simulink model "ctrl_custom_4corner_automatic"  (R2016b)
settings: Solver=ode4  StartTime=0.0  StopTime=inf  FixedStep=0.01  RelTol=1e-3  EnableMultiTasking=on
values from neighbouring files (symbols this model uses):
  alpha = R_T*Eta_t_dot - K1*z_1    [Immersion.m]
undefined symbols (not defined in the file or in its folder): T_pinv_m
libraries: marine_gnc x6, simulink x1
(part 1 of 5)
settings Model: Creator=mclab  LastModifiedBy=utente
settings DataIOCC: LimitDataPoints=on  SaveFormat=Array
settings OptimizationCC: LifeSpan=inf
settings DebuggingCC: SolverPrmCheckMsg=warning  InheritedTsInSrcMsg=none  RootOutportRequireBusObject=error  StrictBusMsg=ErrorOnBusTreatedAsVector  SFUnexpectedBacktrackingDiag=warning  SFNoUnconditionalDefaultTransitionDiag=warning  SFExecutionAtInitializationDiag=none
settings HardwareCC: ProdBitPerPointer=32  ProdBitPerSizeT=32  ProdBitPerPtrDiffT=32  ProdLargestAtomicFloat=None  ProdIntDivRoundTo=Undefined  ProdEndianess=Unspecified  ProdWordSize=32  ProdHWDeviceType=32-bit Generic
settings ModelReferenceCC: PropagateSignalLabelsOutOfModel=off
settings RTWCC: SystemTargetFile=NIVeriStand_VxWorks.tlc  TemplateMakefile=NIVeriStand_VxWorks.tmf  Description=NI VeriStand VxWorks Real-Time Target for Release 2007b or later
settings STFCustomTargetCC: GeneratePreprocessorConditionals=Disable all  MatFileLogging=on  MATLABClassNameForMDSCustomization=Simulink.SoftwareTarget.TargetSpecificTriggerConfigurationBase  SystemTargetFile=NIVeriStand_VxWorks.tlc
settings ConfigComp: CovMetricSettings=dw  CovHtmlReporting=on  CovSaveCumulativeToWorkspaceVar=on  CovSaveSingleToWorkspaceVar=on  CovExternalEMLEnable=off  CovSFcnEnable=off

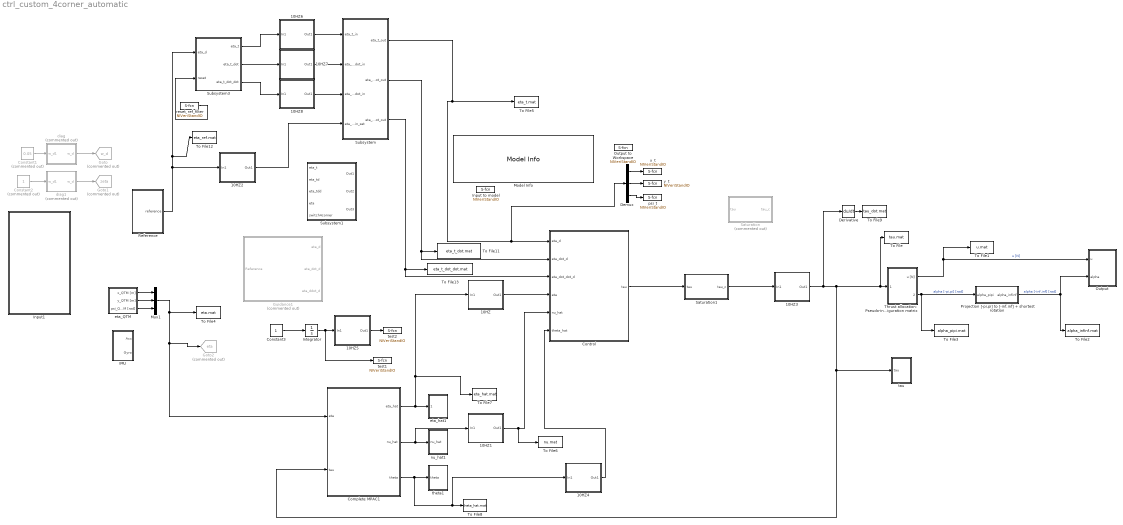
== system ctrl_custom_4corner_automatic ==
  10HZ : Subsystem
  10HZ1 : Subsystem
  10HZ2 : Subsystem
  10HZ3 : Subsystem
  10HZ4 : Subsystem
  10HZ5 : Subsystem
  10HZ6 : Subsystem
  10HZ7 : Subsystem
  10HZ8 : Subsystem
  Complete MPAC1 : Subsystem
  Constant1 : Constant  Commented=on  Value=0.05
  Constant2 : Constant  Commented=on
  Constant3 : Constant
  Control : Subsystem
  Demux : Demux  Outputs=3
  Derivative : Derivative
  Goto : Goto  Commented=on  GotoTag=w_d  TagVisibility=global
  Goto1 : Goto  Commented=on  GotoTag=zeta  TagVisibility=global
  Goto2 : Goto  Commented=on  GotoTag=eta  TagVisibility=global
  Guidance1 : Subsystem  Commented=on
  IMU : Subsystem
  Input to model : S-Function  Priority=1  FunctionName=NIVeriStandIO  Parameters=width dtype portnum stime stype btype  SFunctionDeploymentMode=off  EnableBusSupport=off  mask(NI VeriStand Inport){portnum=1, width=-1, stime=-1, dtype=auto, stype=auto, btype=1}
      mask prompts: portnum "Port number:"; width "Port dimensions (-1 for dynamically sized):"; stime "Sample time (-1 for inherited):"; dtype "Data type:"; stype "Signal type:"; btype "Block type:"
      mask help: Use this inport on any level of nested subsystems to allow NI VeriStand software to map signals to it.
      mask init:
      | NIVeriStandIO_init;
      settings: CopyFcn=NIVeriStand_MDL_functions('', 'IO_copy');  DeleteFcn=NIVeriStand_MDL_functions('', 'IO_delete');  MoveFcn=set_param(gcb, 'Mask', 'on');
      mask Callback portnum: NIVeriStand_MDL_functions('', 'IO_setportnum');
      mask TypeOptions dtype: auto | double | single | int8 | uint8 | int16 | uint16 | int32 | uint32 | boolean
      mask Callback dtype: NIVeriStand_MDL_functions('', 'IO_booleansignal');
      mask TypeOptions stype: auto | real | complex
      mask Display:
      | patch([-x x], [-y y], [.90980 .81960 .32156]);
      | plot([xrad -x x xrad], [yrad -y y yrad]);
      | fprintf('NI In%d', portnum);
  Input1 : Subsystem
  Integrator : Integrator
  Model Info : simulink/Model-Wide Utilities/Model Info  Frame=on  DisplayStringWithTags=|  HorizontalTextAlignment=Center  LeftAlignmentValue=0.5  SourceBlockDiagram=ctrl_custom  TagMaxNumber=20
      | Read me: 
      | In this model you find all the inputs and outputs for controlling CSAD. 
      | DO NOT alter the subsystems IMU, Pose or u. 
      | 
      | For real-time control (e.g. tuning controller gains when the vessel is running) 
      | and monitoring of variables, use NI Veristand Input/Output ports. 
      | You can add as many as you want. Note that these only operates on 
      | single variables, therefore use Mux/Demux/Selector.
      | These variables are accesible from VeriStand Workspace
  Mux1 : Mux  Inputs=3
  Output : Subsystem
  Output to Workspace : S-Function  Priority=1  FunctionName=NIVeriStandIO  Parameters=width dtype portnum stime stype btype  SFunctionDeploymentMode=off  EnableBusSupport=off  mask(NI VeriStand Outport){portnum=1, width=-1, stime=-1, dtype=auto, stype=auto, btype=0}
      mask prompts: portnum "Port number:"; width "Port dimensions (-1 for dynamically sized):"; stime "Sample time (-1 for inherited):"; dtype "Data type:"; stype "Signal type:"; btype "Block type:"
      mask help: Use this outport on any level of nested subsystems to allow NI VeriStand software to map signals to it.
      mask init:
      | NIVeriStandIO_init;
      settings: CopyFcn=NIVeriStand_MDL_functions('', 'IO_copy');  DeleteFcn=NIVeriStand_MDL_functions('', 'IO_delete');  MoveFcn=set_param(gcb, 'Mask', 'on');
      mask Callback portnum: NIVeriStand_MDL_functions('', 'IO_setportnum');
      mask TypeOptions dtype: auto | double | single | int8 | uint8 | int16 | uint16 | int32 | uint32 | boolean
      mask Callback dtype: NIVeriStand_MDL_functions('', 'IO_booleansignal');
      mask TypeOptions stype: auto | real | complex
      mask Display:
      | patch([-x x], [-y y], [.90980 .81960 .32156]);
      | plot([xrad -x x xrad], [yrad -y y yrad]);
      | fprintf('NI Out%d', portnum);
  Projection [-pi,pi] to [-inf,inf] + shortest rotation : Subsystem
  Reference : Subsystem
  Saturation : Subsystem  Commented=on
  Saturation1 : Subsystem
  Subsystem : Subsystem
  Subsystem1 : Subsystem
  Subsystem3 : Subsystem
  Thrust allocation: Pseudo-inverse of extended thrust configuration matrix : Subsystem
  To File : ToFile  Filename=tau.mat  MatrixName=tau
  To File1 : ToFile  Filename=u.mat
  To File11 : ToFile  Filename=eta_t_dot.mat
  To File12 : ToFile  Filename=eta_ref.mat  MatrixName=eta_t
  To File13 : ToFile  Filename=eta_t_dot_dot.mat
  To File2 : ToFile  Filename=alpha_infinf.mat
  To File3 : ToFile  Filename=alpha_pipi.mat
  To File4 : ToFile  Filename=eta.mat  MatrixName=eta
  To File5 : ToFile  Filename=eta_t.mat
  To File6 : ToFile  Filename=nu.mat  MatrixName=nu
  To File7 : ToFile  Filename=eta_hat.mat
  To File8 : ToFile  Filename=theta_hat.mat
  To File9 : ToFile  Filename=tau_dot.mat  MatrixName=tau_dot
  diag : MATLAB Function  Commented=on  TreatAsAtomicUnit=on
  diag1 : MATLAB Function  Commented=on  TreatAsAtomicUnit=on
  eta_QTM : Subsystem
  eta_hat1 : Subsystem
  nu_hat1 : Subsystem
  psi_t : S-Function  Priority=4  FunctionName=NIVeriStandIO  Parameters=width dtype portnum stime stype btype  SFunctionDeploymentMode=off  EnableBusSupport=off  mask(NI VeriStand Outport){portnum=4, width=-1, stime=-1, dtype=auto, stype=auto, btype=0}
      mask prompts: portnum "Port number:"; width "Port dimensions (-1 for dynamically sized):"; stime "Sample time (-1 for inherited):"; dtype "Data type:"; stype "Signal type:"; btype "Block type:"
      mask help: Use this outport on any level of nested subsystems to allow NI VeriStand software to map signals to it.
      mask init:
      | NIVeriStandIO_init;
      settings: CopyFcn=NIVeriStand_MDL_functions('', 'IO_copy');  DeleteFcn=NIVeriStand_MDL_functions('', 'IO_delete');  MoveFcn=set_param(gcb, 'Mask', 'on');
      mask Callback portnum: NIVeriStand_MDL_functions('', 'IO_setportnum');
      mask TypeOptions dtype: auto | double | single | int8 | uint8 | int16 | uint16 | int32 | uint32 | boolean
      mask Callback dtype: NIVeriStand_MDL_functions('', 'IO_booleansignal');
      mask TypeOptions stype: auto | real | complex
      mask Display:
      | patch([-x x], [-y y], [.90980 .81960 .32156]);
      | plot([xrad -x x xrad], [yrad -y y yrad]);
      | fprintf('NI Out%d', portnum);
  reset_ref_filter : S-Function  Priority=2  FunctionName=NIVeriStandIO  Parameters=width dtype portnum stime stype btype  SFunctionDeploymentMode=off  EnableBusSupport=off  mask(NI VeriStand Inport){portnum=2, width=-1, stime=-1, dtype=auto, stype=auto, btype=1}
      mask prompts: portnum "Port number:"; width "Port dimensions (-1 for dynamically sized):"; stime "Sample time (-1 for inherited):"; dtype "Data type:"; stype "Signal type:"; btype "Block type:"
      mask help: Use this inport on any level of nested subsystems to allow NI VeriStand software to map signals to it.
      mask init:
      | NIVeriStandIO_init;
      settings: CopyFcn=NIVeriStand_MDL_functions('', 'IO_copy');  DeleteFcn=NIVeriStand_MDL_functions('', 'IO_delete');  MoveFcn=set_param(gcb, 'Mask', 'on');
      mask Callback portnum: NIVeriStand_MDL_functions('', 'IO_setportnum');
      mask TypeOptions dtype: auto | double | single | int8 | uint8 | int16 | uint16 | int32 | uint32 | boolean
      mask Callback dtype: NIVeriStand_MDL_functions('', 'IO_booleansignal');
      mask TypeOptions stype: auto | real | complex
      mask Display:
      | patch([-x x], [-y y], [.90980 .81960 .32156]);
      | plot([xrad -x x xrad], [yrad -y y yrad]);
      | fprintf('NI In%d', portnum);
  tau : Subsystem
  test1 : S-Function  Priority=6  FunctionName=NIVeriStandIO  Parameters=width dtype portnum stime stype btype  SFunctionDeploymentMode=off  EnableBusSupport=off  mask(NI VeriStand Outport){portnum=6, width=-1, stime=-1, dtype=auto, stype=auto, btype=0}
      mask prompts: portnum "Port number:"; width "Port dimensions (-1 for dynamically sized):"; stime "Sample time (-1 for inherited):"; dtype "Data type:"; stype "Signal type:"; btype "Block type:"
      mask help: Use this outport on any level of nested subsystems to allow NI VeriStand software to map signals to it.
      mask init:
      | NIVeriStandIO_init;
      settings: CopyFcn=NIVeriStand_MDL_functions('', 'IO_copy');  DeleteFcn=NIVeriStand_MDL_functions('', 'IO_delete');  MoveFcn=set_param(gcb, 'Mask', 'on');
      mask Callback portnum: NIVeriStand_MDL_functions('', 'IO_setportnum');
      mask TypeOptions dtype: auto | double | single | int8 | uint8 | int16 | uint16 | int32 | uint32 | boolean
      mask Callback dtype: NIVeriStand_MDL_functions('', 'IO_booleansignal');
      mask TypeOptions stype: auto | real | complex
      mask Display:
      | patch([-x x], [-y y], [.90980 .81960 .32156]);
      | plot([xrad -x x xrad], [yrad -y y yrad]);
      | fprintf('NI Out%d', portnum);
  test2 : S-Function  Priority=5  FunctionName=NIVeriStandIO  Parameters=width dtype portnum stime stype btype  SFunctionDeploymentMode=off  EnableBusSupport=off  mask(NI VeriStand Outport){portnum=5, width=-1, stime=-1, dtype=auto, stype=auto, btype=0}
      mask prompts: portnum "Port number:"; width "Port dimensions (-1 for dynamically sized):"; stime "Sample time (-1 for inherited):"; dtype "Data type:"; stype "Signal type:"; btype "Block type:"
      mask help: Use this outport on any level of nested subsystems to allow NI VeriStand software to map signals to it.
      mask init:
      | NIVeriStandIO_init;
      settings: CopyFcn=NIVeriStand_MDL_functions('', 'IO_copy');  DeleteFcn=NIVeriStand_MDL_functions('', 'IO_delete');  MoveFcn=set_param(gcb, 'Mask', 'on');
      mask Callback portnum: NIVeriStand_MDL_functions('', 'IO_setportnum');
      mask TypeOptions dtype: auto | double | single | int8 | uint8 | int16 | uint16 | int32 | uint32 | boolean
      mask Callback dtype: NIVeriStand_MDL_functions('', 'IO_booleansignal');
      mask TypeOptions stype: auto | real | complex
      mask Display:
      | patch([-x x], [-y y], [.90980 .81960 .32156]);
      | plot([xrad -x x xrad], [yrad -y y yrad]);
      | fprintf('NI Out%d', portnum);
  theta1 : Subsystem
  x_t : S-Function  Priority=2  FunctionName=NIVeriStandIO  Parameters=width dtype portnum stime stype btype  SFunctionDeploymentMode=off  EnableBusSupport=off  mask(NI VeriStand Outport){portnum=2, width=-1, stime=-1, dtype=auto, stype=auto, btype=0}
      mask prompts: portnum "Port number:"; width "Port dimensions (-1 for dynamically sized):"; stime "Sample time (-1 for inherited):"; dtype "Data type:"; stype "Signal type:"; btype "Block type:"
      mask help: Use this outport on any level of nested subsystems to allow NI VeriStand software to map signals to it.
      mask init:
      | NIVeriStandIO_init;
      settings: CopyFcn=NIVeriStand_MDL_functions('', 'IO_copy');  DeleteFcn=NIVeriStand_MDL_functions('', 'IO_delete');  MoveFcn=set_param(gcb, 'Mask', 'on');
      mask Callback portnum: NIVeriStand_MDL_functions('', 'IO_setportnum');
      mask TypeOptions dtype: auto | double | single | int8 | uint8 | int16 | uint16 | int32 | uint32 | boolean
      mask Callback dtype: NIVeriStand_MDL_functions('', 'IO_booleansignal');
      mask TypeOptions stype: auto | real | complex
      mask Display:
      | patch([-x x], [-y y], [.90980 .81960 .32156]);
      | plot([xrad -x x xrad], [yrad -y y yrad]);
      | fprintf('NI Out%d', portnum);
  y_t : S-Function  Priority=3  FunctionName=NIVeriStandIO  Parameters=width dtype portnum stime stype btype  SFunctionDeploymentMode=off  EnableBusSupport=off  mask(NI VeriStand Outport){portnum=3, width=-1, stime=-1, dtype=auto, stype=auto, btype=0}
      mask prompts: portnum "Port number:"; width "Port dimensions (-1 for dynamically sized):"; stime "Sample time (-1 for inherited):"; dtype "Data type:"; stype "Signal type:"; btype "Block type:"
      mask help: Use this outport on any level of nested subsystems to allow NI VeriStand software to map signals to it.
      mask init:
      | NIVeriStandIO_init;
      settings: CopyFcn=NIVeriStand_MDL_functions('', 'IO_copy');  DeleteFcn=NIVeriStand_MDL_functions('', 'IO_delete');  MoveFcn=set_param(gcb, 'Mask', 'on');
      mask Callback portnum: NIVeriStand_MDL_functions('', 'IO_setportnum');
      mask TypeOptions dtype: auto | double | single | int8 | uint8 | int16 | uint16 | int32 | uint32 | boolean
      mask Callback dtype: NIVeriStand_MDL_functions('', 'IO_booleansignal');
      mask TypeOptions stype: auto | real | complex
      mask Display:
      | patch([-x x], [-y y], [.90980 .81960 .32156]);
      | plot([xrad -x x xrad], [yrad -y y yrad]);
      | fprintf('NI Out%d', portnum);
  wires:
  Thrust allocation: Pseudo-inverse of extended thrust configuration matrix/1(u [N]) -> Output/1(u), To File1/1  "u [N]"
  Thrust allocation: Pseudo-inverse of extended thrust configuration matrix/2(alpha [rad]) -> To File3/1, Projection [-pi,pi] to [-inf,inf] + shortest rotation/1(alpha_pipi)  "alpha [-pi,pi] [rad]"
  Projection [-pi,pi] to [-inf,inf] + shortest rotation/1(alpha_infinf) -> Output/2(alpha), To File2/1  "alpha [-inf,inf] [rad]"
  eta_QTM/1(x_QTM [m]) -> Mux1/1
  eta_QTM/2(y_QTM [m]) -> Mux1/2
  eta_QTM/3(psi_QTM [rad]) -> Mux1/3
  Demux/1 -> x_t/1
  Demux/2 -> y_t/1
  Demux/3 -> psi_t/1
  Constant1/1 -> diag/1(w_d1)
  Constant2/1 -> diag1/1(w_d1)
  diag/1(w_d) -> Goto/1
  diag1/1(w_d) -> Goto1/1
  Reference/1(reference) -> To File12/1, Subsystem3/1(eta_d), 10HZ2/1(In1)
  Constant3/1 -> Integrator/1
  Integrator/1 -> test1/1, 10HZ5/1(In1)
  Complete MPAC1/2(nu_hat) -> 10HZ1/1(In1), nu_hat1/1(nu_hat)
  Complete MPAC1/3(theta) -> 10HZ4/1(In1), To File8/1, theta1/1(theta)
  Complete MPAC1/1(eta_hat) -> To File7/1, 10HZ/1(In1), eta_hat1/1(eta_hat)
  Mux1/1 -> Complete MPAC1/1(eta), Goto2/1, To File4/1
  10HZ/1(Out1) -> Control/4(eta)
  10HZ1/1(Out1) -> To File6/1, Control/5(nu_hat)
  10HZ3/1(Out1) -> Derivative/1, Thrust allocation: Pseudo-inverse of extended thrust configuration matrix/1(tau [N]), To File/1, Complete MPAC1/2(tau), tau/1(tau)
  10HZ4/1(Out1) -> Control/6(theta_hat)
  10HZ5/1(Out1) -> test2/1
  Subsystem3/1(eta_t) -> 10HZ6/1(In1)
  Subsystem3/2(eta_t_dot) -> 10HZ7/1(In1)
  Subsystem3/3(eta_t_dot_dot) -> 10HZ8/1(In1)
  Subsystem/1(eta_t_out) -> Demux/1, Control/1(eta_d), To File5/1
  10HZ6/1(Out1) -> Subsystem/1(eta_t_in)
  10HZ7/1(Out1) -> Subsystem/2(eta_t_dot_in)
  10HZ8/1(Out1) -> Subsystem/3(eta_t_dot_dot_in)
  10HZ2/1(Out1) -> Subsystem/4(eta_t_in_set)
  Subsystem/2(eta_t_dot_out) -> To File11/1, Control/2(eta_dot_d)
  Subsystem/3(eta_t_dot_dot_out) -> To File13/1, Control/3(eta_dot_dot_d)
  reset_ref_filter/1 -> Subsystem3/2(reset)
  Control/1(tau) -> Saturation1/1(tau)
  Saturation1/1(tau_c) -> 10HZ3/1(In1)
  Derivative/1 -> To File9/1

== system ctrl_custom_4corner_automatic/10HZ ==
  In1 : Inport
  MATLAB Function : MATLAB Function  TreatAsAtomicUnit=on
  Memory : Memory
  Memory1 : Memory
  Out1 : Outport
  wires:
  Memory/1 -> MATLAB Function/3(i)
  MATLAB Function/2(i_out) -> Memory/1
  Memory1/1 -> MATLAB Function/2(nu_current)
  MATLAB Function/1(nu_10) -> Out1/1, Memory1/1
  In1/1 -> MATLAB Function/1(nu)

== system ctrl_custom_4corner_automatic/10HZ1 ==
  In1 : Inport
  MATLAB Function : MATLAB Function  TreatAsAtomicUnit=on
  Memory : Memory
  Memory1 : Memory
  Out1 : Outport
  wires:
  Memory/1 -> MATLAB Function/3(i)
  MATLAB Function/2(i_out) -> Memory/1
  Memory1/1 -> MATLAB Function/2(nu_current)
  MATLAB Function/1(nu_10) -> Out1/1, Memory1/1
  In1/1 -> MATLAB Function/1(nu)

== system ctrl_custom_4corner_automatic/10HZ2 ==
  In1 : Inport
  MATLAB Function : MATLAB Function  TreatAsAtomicUnit=on
  Memory : Memory
  Memory1 : Memory
  Out1 : Outport
  wires:
  Memory/1 -> MATLAB Function/3(i)
  MATLAB Function/2(i_out) -> Memory/1
  Memory1/1 -> MATLAB Function/2(nu_current)
  MATLAB Function/1(nu_10) -> Out1/1, Memory1/1
  In1/1 -> MATLAB Function/1(nu)

== system ctrl_custom_4corner_automatic/10HZ3 ==
  In1 : Inport
  MATLAB Function : MATLAB Function  TreatAsAtomicUnit=on
  Memory : Memory
  Memory1 : Memory
  Out1 : Outport
  wires:
  In1/1 -> MATLAB Function/1(nu)
  MATLAB Function/1(nu_10) -> Memory1/1, Out1/1
  Memory1/1 -> MATLAB Function/2(nu_current)
  MATLAB Function/2(i_out) -> Memory/1
  Memory/1 -> MATLAB Function/3(i)

== system ctrl_custom_4corner_automatic/10HZ4 ==
  In1 : Inport
  MATLAB Function : MATLAB Function  TreatAsAtomicUnit=on
  Memory : Memory
  Memory1 : Memory
  Out1 : Outport
  wires:
  In1/1 -> MATLAB Function/1(nu)
  MATLAB Function/1(nu_10) -> Memory1/1, Out1/1
  Memory1/1 -> MATLAB Function/2(nu_current)
  MATLAB Function/2(i_out) -> Memory/1
  Memory/1 -> MATLAB Function/3(i)

== system ctrl_custom_4corner_automatic/10HZ5 ==
  In1 : Inport
  MATLAB Function : MATLAB Function  TreatAsAtomicUnit=on
  Memory : Memory
  Memory1 : Memory
  Out1 : Outport
  wires:
  Memory/1 -> MATLAB Function/3(i)
  MATLAB Function/2(i_out) -> Memory/1
  Memory1/1 -> MATLAB Function/2(nu_current)
  MATLAB Function/1(nu_10) -> Out1/1, Memory1/1
  In1/1 -> MATLAB Function/1(nu)

== system ctrl_custom_4corner_automatic/10HZ6 ==
  In1 : Inport
  MATLAB Function : MATLAB Function  TreatAsAtomicUnit=on
  Memory : Memory
  Memory1 : Memory
  Out1 : Outport
  wires:
  In1/1 -> MATLAB Function/1(nu)
  MATLAB Function/1(nu_10) -> Memory1/1, Out1/1
  Memory1/1 -> MATLAB Function/2(nu_current)
  MATLAB Function/2(i_out) -> Memory/1
  Memory/1 -> MATLAB Function/3(i)

== system ctrl_custom_4corner_automatic/10HZ7 ==
  In1 : Inport
  MATLAB Function : MATLAB Function  TreatAsAtomicUnit=on
  Memory : Memory
  Memory1 : Memory
  Out1 : Outport
  wires:
  In1/1 -> MATLAB Function/1(nu)
  MATLAB Function/1(nu_10) -> Memory1/1, Out1/1
  Memory1/1 -> MATLAB Function/2(nu_current)
  MATLAB Function/2(i_out) -> Memory/1
  Memory/1 -> MATLAB Function/3(i)

== system ctrl_custom_4corner_automatic/10HZ8 ==
  In1 : Inport
  MATLAB Function : MATLAB Function  TreatAsAtomicUnit=on
  Memory : Memory
  Memory1 : Memory
  Out1 : Outport
  wires:
  Memory/1 -> MATLAB Function/3(i)
  MATLAB Function/2(i_out) -> Memory/1
  Memory1/1 -> MATLAB Function/2(nu_current)
  MATLAB Function/1(nu_10) -> Out1/1, Memory1/1
  In1/1 -> MATLAB Function/1(nu)

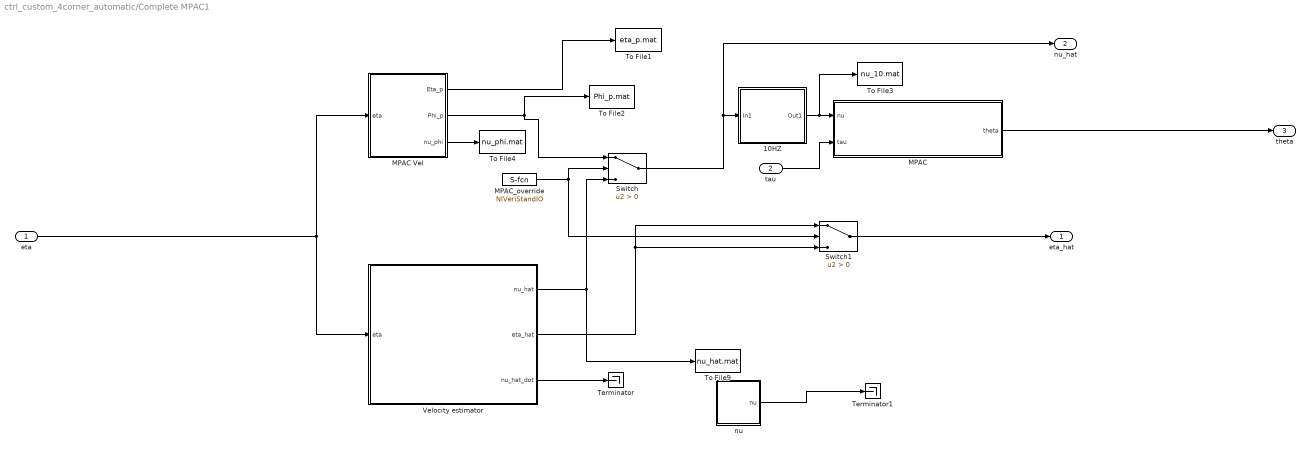
== system ctrl_custom_4corner_automatic/Complete MPAC1 ==
  eta : Inport
  tau : Inport  Port=2
  10HZ : Subsystem
  MPAC : Subsystem
  MPAC Vel : Subsystem
  MPAC_override : S-Function  Priority=1  FunctionName=NIVeriStandIO  Parameters=width dtype portnum stime stype btype  SFunctionDeploymentMode=off  EnableBusSupport=off  mask(NI VeriStand Inport){portnum=1, width=-1, stime=-1, dtype=auto, stype=auto, btype=1}
      mask prompts: portnum "Port number:"; width "Port dimensions (-1 for dynamically sized):"; stime "Sample time (-1 for inherited):"; dtype "Data type:"; stype "Signal type:"; btype "Block type:"
      mask help: Use this inport on any level of nested subsystems to allow NI VeriStand software to map signals to it.
      mask init:
      | NIVeriStandIO_init;
      settings: CopyFcn=NIVeriStand_MDL_functions('', 'IO_copy');  DeleteFcn=NIVeriStand_MDL_functions('', 'IO_delete');  MoveFcn=set_param(gcb, 'Mask', 'on');
      mask Callback portnum: NIVeriStand_MDL_functions('', 'IO_setportnum');
      mask TypeOptions dtype: auto | double | single | int8 | uint8 | int16 | uint16 | int32 | uint32 | boolean
      mask Callback dtype: NIVeriStand_MDL_functions('', 'IO_booleansignal');
      mask TypeOptions stype: auto | real | complex
      mask Display:
      | patch([-x x], [-y y], [.90980 .81960 .32156]);
      | plot([xrad -x x xrad], [yrad -y y yrad]);
      | fprintf('NI In%d', portnum);
  Switch : Switch  Criteria=u2 > Threshold
  Switch1 : Switch  Criteria=u2 > Threshold
  Terminator : Terminator
  Terminator1 : Terminator
  To File1 : ToFile  Filename=eta_p.mat
  To File2 : ToFile  Filename=Phi_p.mat
  To File3 : ToFile  Filename=nu_10.mat
  To File4 : ToFile  Filename=nu_phi.mat
  To File9 : ToFile  Filename=nu_hat.mat
  Velocity estimator : Subsystem
  nu : Subsystem
  eta_hat : Outport
  nu_hat : Outport  Port=2
  theta : Outport  Port=3
  wires:
  MPAC Vel/2(Phi_p) -> Switch/1, To File2/1
  Velocity estimator/1(nu_hat) -> To File9/1, Switch/3
  MPAC_override/1 -> Switch1/2, Switch/2
  eta/1 -> MPAC Vel/1(eta), Velocity estimator/1(eta)
  tau/1 -> MPAC/2(tau)
  Velocity estimator/2(eta_hat) -> Switch1/1, Switch1/3
  MPAC/1(theta) -> theta/1
  MPAC Vel/1(Eta_p) -> To File1/1
  Switch1/1 -> eta_hat/1
  Velocity estimator/3(nu_hat_dot) -> Terminator/1
  Switch/1 -> 10HZ/1(In1), nu_hat/1
  nu/1(nu) -> Terminator1/1
  10HZ/1(Out1) -> To File3/1, MPAC/1(nu)
  MPAC Vel/3(nu_phi) -> To File4/1

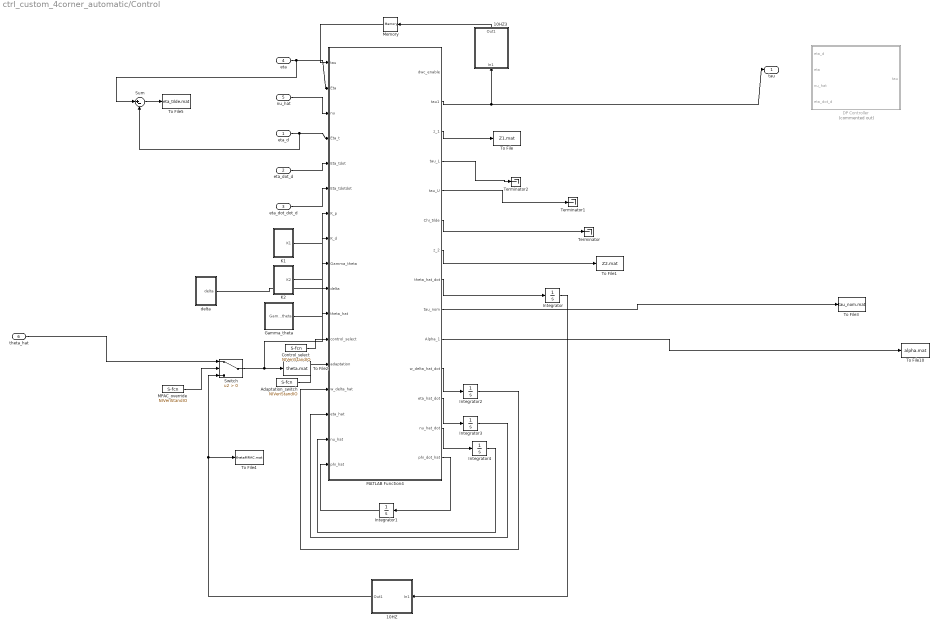
== system ctrl_custom_4corner_automatic/Control ==
  eta_d : Inport
  eta_dot_d : Inport  Port=2
  eta_dot_dot_d : Inport  Port=3
  eta : Inport  Port=4
  nu_hat : Inport  Port=5
  theta_hat : Inport  Port=6
  10HZ : Subsystem
  10HZ3 : Subsystem
  Adaptation_switch : S-Function  Priority=1  FunctionName=NIVeriStandIO  Parameters=width dtype portnum stime stype btype  SFunctionDeploymentMode=off  EnableBusSupport=off  mask(NI VeriStand Inport){portnum=1, width=-1, stime=-1, dtype=auto, stype=auto, btype=1}
      mask prompts: portnum "Port number:"; width "Port dimensions (-1 for dynamically sized):"; stime "Sample time (-1 for inherited):"; dtype "Data type:"; stype "Signal type:"; btype "Block type:"
      mask help: Use this inport on any level of nested subsystems to allow NI VeriStand software to map signals to it.
      mask init:
      | NIVeriStandIO_init;
      settings: CopyFcn=NIVeriStand_MDL_functions('', 'IO_copy');  DeleteFcn=NIVeriStand_MDL_functions('', 'IO_delete');  MoveFcn=set_param(gcb, 'Mask', 'on');
      mask Callback portnum: NIVeriStand_MDL_functions('', 'IO_setportnum');
      mask TypeOptions dtype: auto | double | single | int8 | uint8 | int16 | uint16 | int32 | uint32 | boolean
      mask Callback dtype: NIVeriStand_MDL_functions('', 'IO_booleansignal');
      mask TypeOptions stype: auto | real | complex
      mask Display:
      | patch([-x x], [-y y], [.90980 .81960 .32156]);
      | plot([xrad -x x xrad], [yrad -y y yrad]);
      | fprintf('NI In%d', portnum);
  Control_select : S-Function  Priority=3  FunctionName=NIVeriStandIO  Parameters=width dtype portnum stime stype btype  SFunctionDeploymentMode=off  EnableBusSupport=off  mask(NI VeriStand Inport){portnum=3, width=-1, stime=-1, dtype=auto, stype=auto, btype=1}
      mask prompts: portnum "Port number:"; width "Port dimensions (-1 for dynamically sized):"; stime "Sample time (-1 for inherited):"; dtype "Data type:"; stype "Signal type:"; btype "Block type:"
      mask help: Use this inport on any level of nested subsystems to allow NI VeriStand software to map signals to it.
      mask init:
      | NIVeriStandIO_init;
      settings: CopyFcn=NIVeriStand_MDL_functions('', 'IO_copy');  DeleteFcn=NIVeriStand_MDL_functions('', 'IO_delete');  MoveFcn=set_param(gcb, 'Mask', 'on');
      mask Callback portnum: NIVeriStand_MDL_functions('', 'IO_setportnum');
      mask TypeOptions dtype: auto | double | single | int8 | uint8 | int16 | uint16 | int32 | uint32 | boolean
      mask Callback dtype: NIVeriStand_MDL_functions('', 'IO_booleansignal');
      mask TypeOptions stype: auto | real | complex
      mask Display:
      | patch([-x x], [-y y], [.90980 .81960 .32156]);
      | plot([xrad -x x xrad], [yrad -y y yrad]);
      | fprintf('NI In%d', portnum);
  DP Controller : Subsystem  Commented=on
  Gamma_theta : Subsystem
  Integrator{,2..4} (4 alike) : Integrator  InitialCondition=[0 0 0]
  Integrator1 : Integrator
  K1 : Subsystem
  K2 : Subsystem
  MATLAB Function4 : MATLAB Function  TreatAsAtomicUnit=on
  MPAC_override : S-Function  Priority=2  FunctionName=NIVeriStandIO  Parameters=width dtype portnum stime stype btype  SFunctionDeploymentMode=off  EnableBusSupport=off  mask(NI VeriStand Inport){portnum=2, width=-1, stime=-1, dtype=auto, stype=auto, btype=1}
      mask prompts: portnum "Port number:"; width "Port dimensions (-1 for dynamically sized):"; stime "Sample time (-1 for inherited):"; dtype "Data type:"; stype "Signal type:"; btype "Block type:"
      mask help: Use this inport on any level of nested subsystems to allow NI VeriStand software to map signals to it.
      mask init:
      | NIVeriStandIO_init;
      settings: CopyFcn=NIVeriStand_MDL_functions('', 'IO_copy');  DeleteFcn=NIVeriStand_MDL_functions('', 'IO_delete');  MoveFcn=set_param(gcb, 'Mask', 'on');
      mask Callback portnum: NIVeriStand_MDL_functions('', 'IO_setportnum');
      mask TypeOptions dtype: auto | double | single | int8 | uint8 | int16 | uint16 | int32 | uint32 | boolean
      mask Callback dtype: NIVeriStand_MDL_functions('', 'IO_booleansignal');
      mask TypeOptions stype: auto | real | complex
      mask Display:
      | patch([-x x], [-y y], [.90980 .81960 .32156]);
      | plot([xrad -x x xrad], [yrad -y y yrad]);
      | fprintf('NI In%d', portnum);
  Memory : Memory  X0=[0 0 0]'
  Sum : Sum  Inputs=|+-
  Switch : Switch  Criteria=u2 > Threshold
  Terminator : Terminator
  Terminator1 : Terminator
  Terminator2 : Terminator
  To File : ToFile  Filename=Z1.mat
  To File1 : ToFile  Filename=Z2.mat
  To File10 : ToFile  Filename=alpha.mat  MatrixName=alpha
  To File2 : ToFile  Filename=theta.mat
  To File3 : ToFile  Filename=tau_nom.mat
  To File4 : ToFile  Filename=thetaMRAC.mat
  To File5 : ToFile  Filename=eta_tilde.mat
  delta : Subsystem
  tau : Outport
  wires:
  eta_dot_d/1 -> MATLAB Function4/5(Eta_tdot)
  eta/1 -> Sum/1, MATLAB Function4/2(Eta)
  nu_hat/1 -> MATLAB Function4/3(nu)
  eta_dot_dot_d/1 -> MATLAB Function4/6(Eta_tdotdot)
  MATLAB Function4/7(z_2) -> To File1/1
  eta_d/1 -> Sum/2, MATLAB Function4/4(Eta_t)
  MATLAB Function4/3(z_1) -> To File/1
  delta/1(delta) -> MATLAB Function4/10(delta)
  K1/1(K1) -> MATLAB Function4/7(K_p)
  K2/1(K2) -> MATLAB Function4/8(K_d)
  Adaptation_switch/1 -> MATLAB Function4/13(adaptation)
  MATLAB Function4/8(theta_hat_dot) -> Integrator/1
  Switch/1 -> MATLAB Function4/11(theta_hat), To File2/1
  MPAC_override/1 -> Switch/2
  Integrator/1 -> 10HZ/1(In1)
  Control_select/1 -> MATLAB Function4/12(control_select)
  MATLAB Function4/5(tau_U) -> Terminator1/1
  MATLAB Function4/6(Chi_tilde) -> Terminator/1
  MATLAB Function4/4(tau_L) -> Terminator2/1
  Gamma_theta/1(Gamma_theta) -> MATLAB Function4/9(Gamma_theta)
  MATLAB Function4/9(tau_nom) -> To File3/1
  10HZ/1(Out1) -> To File4/1, Switch/3
  theta_hat/1 -> Switch/1
  Sum/1 -> To File5/1
  MATLAB Function4/2(tau1) -> tau/1, 10HZ3/1(In1)
  MATLAB Function4/10(Alpha_1) -> To File10/1
  Memory/1 -> MATLAB Function4/1(tau)
  MATLAB Function4/11(w_delta_hat_dot) -> Integrator2/1
  MATLAB Function4/12(eta_hat_dot) -> Integrator3/1
  MATLAB Function4/13(nu_hat_dot) -> Integrator4/1
  Integrator4/1 -> MATLAB Function4/16(nu_hat)
  Integrator3/1 -> MATLAB Function4/15(eta_hat)
  Integrator2/1 -> MATLAB Function4/14(w_delta_hat)
  10HZ3/1(Out1) -> Memory/1
  Integrator1/1 -> MATLAB Function4/17(phi_hat)
  MATLAB Function4/14(phi_dot_hat) -> Integrator1/1

== system ctrl_custom_4corner_automatic/Guidance1 ==
  "Reference " : Inport
  Reference model : Subsystem
  eta_d : Outport
  eta_dot_d : Outport  Port=2
  eta_ddot_d : Outport  Port=3
  wires:
  Reference model/1(eta_d) -> eta_d/1
  Reference model/2(eta_dot_d) -> eta_dot_d/1
  Reference model/3(eta_ddot_d) -> eta_ddot_d/1
  "Reference "/1 -> Reference model/1(reference)

== system ctrl_custom_4corner_automatic/IMU ==
  note: Measurement in deg/s
  note: Measurement in g
  Acc_x : S-Function  Priority=1  FunctionName=NIVeriStandIO  Parameters=width dtype portnum stime stype btype  SFunctionDeploymentMode=off  EnableBusSupport=off  mask(NI VeriStand Inport){portnum=1, width=-1, stime=-1, dtype=auto, stype=auto, btype=1}
      mask prompts: portnum "Port number:"; width "Port dimensions (-1 for dynamically sized):"; stime "Sample time (-1 for inherited):"; dtype "Data type:"; stype "Signal type:"; btype "Block type:"
      mask help: Use this inport on any level of nested subsystems to allow NI VeriStand software to map signals to it.
      mask init:
      | NIVeriStandIO_init;
      settings: CopyFcn=NIVeriStand_MDL_functions('', 'IO_copy');  DeleteFcn=NIVeriStand_MDL_functions('', 'IO_delete');  MoveFcn=set_param(gcb, 'Mask', 'on');
      mask Callback portnum: NIVeriStand_MDL_functions('', 'IO_setportnum');
      mask TypeOptions dtype: auto | double | single | int8 | uint8 | int16 | uint16 | int32 | uint32 | boolean
      mask Callback dtype: NIVeriStand_MDL_functions('', 'IO_booleansignal');
      mask TypeOptions stype: auto | real | complex
      mask Display:
      | patch([-x x], [-y y], [.90980 .81960 .32156]);
      | plot([xrad -x x xrad], [yrad -y y yrad]);
      | fprintf('NI In%d', portnum);
  Acc_y : S-Function  Priority=2  FunctionName=NIVeriStandIO  Parameters=width dtype portnum stime stype btype  SFunctionDeploymentMode=off  EnableBusSupport=off  mask(NI VeriStand Inport){portnum=2, width=-1, stime=-1, dtype=auto, stype=auto, btype=1}
      mask prompts: portnum "Port number:"; width "Port dimensions (-1 for dynamically sized):"; stime "Sample time (-1 for inherited):"; dtype "Data type:"; stype "Signal type:"; btype "Block type:"
      mask help: Use this inport on any level of nested subsystems to allow NI VeriStand software to map signals to it.
      mask init:
      | NIVeriStandIO_init;
      settings: CopyFcn=NIVeriStand_MDL_functions('', 'IO_copy');  DeleteFcn=NIVeriStand_MDL_functions('', 'IO_delete');  MoveFcn=set_param(gcb, 'Mask', 'on');
      mask Callback portnum: NIVeriStand_MDL_functions('', 'IO_setportnum');
      mask TypeOptions dtype: auto | double | single | int8 | uint8 | int16 | uint16 | int32 | uint32 | boolean
      mask Callback dtype: NIVeriStand_MDL_functions('', 'IO_booleansignal');
      mask TypeOptions stype: auto | real | complex
      mask Display:
      | patch([-x x], [-y y], [.90980 .81960 .32156]);
      | plot([xrad -x x xrad], [yrad -y y yrad]);
      | fprintf('NI In%d', portnum);
  Acc_z : S-Function  Priority=3  FunctionName=NIVeriStandIO  Parameters=width dtype portnum stime stype btype  SFunctionDeploymentMode=off  EnableBusSupport=off  mask(NI VeriStand Inport){portnum=3, width=-1, stime=-1, dtype=auto, stype=auto, btype=1}
      mask prompts: portnum "Port number:"; width "Port dimensions (-1 for dynamically sized):"; stime "Sample time (-1 for inherited):"; dtype "Data type:"; stype "Signal type:"; btype "Block type:"
      mask help: Use this inport on any level of nested subsystems to allow NI VeriStand software to map signals to it.
      mask init:
      | NIVeriStandIO_init;
      settings: CopyFcn=NIVeriStand_MDL_functions('', 'IO_copy');  DeleteFcn=NIVeriStand_MDL_functions('', 'IO_delete');  MoveFcn=set_param(gcb, 'Mask', 'on');
      mask Callback portnum: NIVeriStand_MDL_functions('', 'IO_setportnum');
      mask TypeOptions dtype: auto | double | single | int8 | uint8 | int16 | uint16 | int32 | uint32 | boolean
      mask Callback dtype: NIVeriStand_MDL_functions('', 'IO_booleansignal');
      mask TypeOptions stype: auto | real | complex
      mask Display:
      | patch([-x x], [-y y], [.90980 .81960 .32156]);
      | plot([xrad -x x xrad], [yrad -y y yrad]);
      | fprintf('NI In%d', portnum);
  Gyro_x : S-Function  Priority=4  FunctionName=NIVeriStandIO  Parameters=width dtype portnum stime stype btype  SFunctionDeploymentMode=off  EnableBusSupport=off  mask(NI VeriStand Inport){portnum=4, width=-1, stime=-1, dtype=auto, stype=auto, btype=1}
      mask prompts: portnum "Port number:"; width "Port dimensions (-1 for dynamically sized):"; stime "Sample time (-1 for inherited):"; dtype "Data type:"; stype "Signal type:"; btype "Block type:"
      mask help: Use this inport on any level of nested subsystems to allow NI VeriStand software to map signals to it.
      mask init:
      | NIVeriStandIO_init;
      settings: CopyFcn=NIVeriStand_MDL_functions('', 'IO_copy');  DeleteFcn=NIVeriStand_MDL_functions('', 'IO_delete');  MoveFcn=set_param(gcb, 'Mask', 'on');
      mask Callback portnum: NIVeriStand_MDL_functions('', 'IO_setportnum');
      mask TypeOptions dtype: auto | double | single | int8 | uint8 | int16 | uint16 | int32 | uint32 | boolean
      mask Callback dtype: NIVeriStand_MDL_functions('', 'IO_booleansignal');
      mask TypeOptions stype: auto | real | complex
      mask Display:
      | patch([-x x], [-y y], [.90980 .81960 .32156]);
      | plot([xrad -x x xrad], [yrad -y y yrad]);
      | fprintf('NI In%d', portnum);
  Gyro_y : S-Function  Priority=5  FunctionName=NIVeriStandIO  Parameters=width dtype portnum stime stype btype  SFunctionDeploymentMode=off  EnableBusSupport=off  mask(NI VeriStand Inport){portnum=5, width=-1, stime=-1, dtype=auto, stype=auto, btype=1}
      mask prompts: portnum "Port number:"; width "Port dimensions (-1 for dynamically sized):"; stime "Sample time (-1 for inherited):"; dtype "Data type:"; stype "Signal type:"; btype "Block type:"
      mask help: Use this inport on any level of nested subsystems to allow NI VeriStand software to map signals to it.
      mask init:
      | NIVeriStandIO_init;
      settings: CopyFcn=NIVeriStand_MDL_functions('', 'IO_copy');  DeleteFcn=NIVeriStand_MDL_functions('', 'IO_delete');  MoveFcn=set_param(gcb, 'Mask', 'on');
      mask Callback portnum: NIVeriStand_MDL_functions('', 'IO_setportnum');
      mask TypeOptions dtype: auto | double | single | int8 | uint8 | int16 | uint16 | int32 | uint32 | boolean
      mask Callback dtype: NIVeriStand_MDL_functions('', 'IO_booleansignal');
      mask TypeOptions stype: auto | real | complex
      mask Display:
      | patch([-x x], [-y y], [.90980 .81960 .32156]);
      | plot([xrad -x x xrad], [yrad -y y yrad]);
      | fprintf('NI In%d', portnum);
  Gyro_z : S-Function  Priority=6  FunctionName=NIVeriStandIO  Parameters=width dtype portnum stime stype btype  SFunctionDeploymentMode=off  EnableBusSupport=off  mask(NI VeriStand Inport){portnum=6, width=-1, stime=-1, dtype=auto, stype=auto, btype=1}
      mask prompts: portnum "Port number:"; width "Port dimensions (-1 for dynamically sized):"; stime "Sample time (-1 for inherited):"; dtype "Data type:"; stype "Signal type:"; btype "Block type:"
      mask help: Use this inport on any level of nested subsystems to allow NI VeriStand software to map signals to it.
      mask init:
      | NIVeriStandIO_init;
      settings: CopyFcn=NIVeriStand_MDL_functions('', 'IO_copy');  DeleteFcn=NIVeriStand_MDL_functions('', 'IO_delete');  MoveFcn=set_param(gcb, 'Mask', 'on');
      mask Callback portnum: NIVeriStand_MDL_functions('', 'IO_setportnum');
      mask TypeOptions dtype: auto | double | single | int8 | uint8 | int16 | uint16 | int32 | uint32 | boolean
      mask Callback dtype: NIVeriStand_MDL_functions('', 'IO_booleansignal');
      mask TypeOptions stype: auto | real | complex
      mask Display:
      | patch([-x x], [-y y], [.90980 .81960 .32156]);
      | plot([xrad -x x xrad], [yrad -y y yrad]);
      | fprintf('NI In%d', portnum);
  Mux : Mux  Inputs=3
  Mux1 : Mux  Inputs=3
  Acc : Outport
  Gyro : Outport  Port=2
  wires:
  Acc_x/1 -> Mux/1
  Acc_y/1 -> Mux/2
  Acc_z/1 -> Mux/3
  Gyro_z/1 -> Mux1/3
  Gyro_y/1 -> Mux1/2
  Gyro_x/1 -> Mux1/1
  Mux1/1 -> Gyro/1
  Mux/1 -> Acc/1

== system ctrl_custom_4corner_automatic/Input1 ==
  Control Gains : Subsystem  Commented=on
  Goto3 : Goto  Commented=on  GotoTag=reset  TagVisibility=global
  Guidance gains : Subsystem  Commented=on
  Observer Gains : Subsystem  Commented=on
  reset : S-Function  Priority=1  Commented=on  FunctionName=NIVeriStandIO  Parameters=width dtype portnum stime stype btype  SFunctionDeploymentMode=off  EnableBusSupport=off  mask(NI VeriStand Inport){portnum=1, width=-1, stime=-1, dtype=auto, stype=auto, btype=1}
      mask prompts: portnum "Port number:"; width "Port dimensions (-1 for dynamically sized):"; stime "Sample time (-1 for inherited):"; dtype "Data type:"; stype "Signal type:"; btype "Block type:"
      mask help: Use this inport on any level of nested subsystems to allow NI VeriStand software to map signals to it.
      mask init:
      | NIVeriStandIO_init;
      settings: CopyFcn=NIVeriStand_MDL_functions('', 'IO_copy');  DeleteFcn=NIVeriStand_MDL_functions('', 'IO_delete');  MoveFcn=set_param(gcb, 'Mask', 'on');
      mask Callback portnum: NIVeriStand_MDL_functions('', 'IO_setportnum');
      mask TypeOptions dtype: auto | double | single | int8 | uint8 | int16 | uint16 | int32 | uint32 | boolean
      mask Callback dtype: NIVeriStand_MDL_functions('', 'IO_booleansignal');
      mask TypeOptions stype: auto | real | complex
      mask Display:
      | patch([-x x], [-y y], [.90980 .81960 .32156]);
      | plot([xrad -x x xrad], [yrad -y y yrad]);
      | fprintf('NI In%d', portnum);
  wires:
  reset/1 -> Goto3/1
